simulink model "task_4"  (R2024a)
settings: Solver=VariableStepAuto  StartTime=0.0  StopTime=50  MaxStep=0.001  RelTol=1e-3
undefined symbols (not defined in the file): k
settings Model: Creator=kit  LastModifiedBy=kit

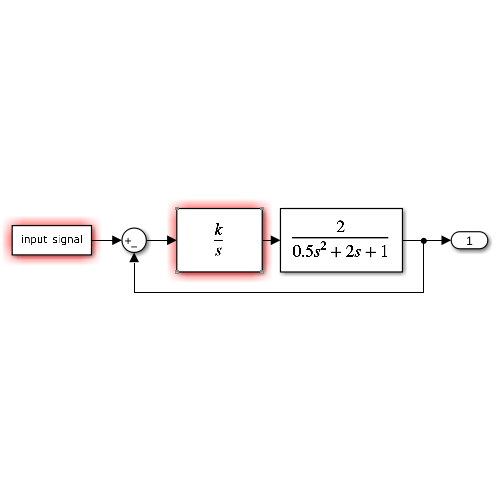
[thumbnail: Simulink's stored preview of the top-level diagram]
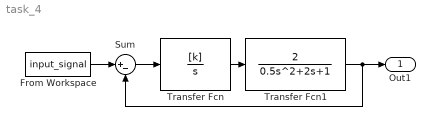
== system task_4 ==
  From Workspace : FromWorkspace  VariableName=input_signal
  Sum : Sum  Inputs=|+-
  Transfer Fcn : TransferFcn  Numerator=[k]  Denominator=[1 0]
  Transfer Fcn1 : TransferFcn  Numerator=[2]  Denominator=[0.5 2 1]
  Out1 : Outport
  wires:
  Sum/1 -> Transfer Fcn/1
  Transfer Fcn/1 -> Transfer Fcn1/1
  Transfer Fcn1/1 -> Sum/2, Out1/1
  From Workspace/1 -> Sum/1
